simulink model "ad9361_tx_filter"  (R2021a)
settings: Solver=ode23tb  StartTime=0.0  StopTime=inf  RelTol=1e-3  EnableMultiTasking=on
PreLoadFcn:
  | ad9361_preload(bdroot,'tx')
  | Fs = 30.72e6
undefined symbols (not defined in the file or in its folder): magnitude
libraries: ad9371_utilities x1, dspmathops x1, dspsrcs4 x1, ad9361_models x1
CloseFcn:
  | clear ad9361_tx_hm1Filt ad9361_tx_hm2Filt;
  | clear ad9361_tx_hm3Filt ad9361_tx_hm4Filt;
settings Model: SimulationMode=accelerator  NumberOfSteps=100  Creator=The MathWorks Inc.  LastModifiedBy=Michael
settings SolverCC: AlgebraicLoopSolver=TrustRegion
settings DataIOCC: ExternalInput=txWaveform  SaveFormat=StructureWithTime  SaveOutput=off  SignalLogging=off  DSMLogging=off  SaveTime=off  ReturnWorkspaceOutputs=off  OutputSaveName=rx
settings OptimizationCC: DefaultParameterBehavior=Inlined  InlineInvariantSignals=on  LifeSpan=inf  SimCompilerOptimization=on
settings DebuggingCC: UnderspecifiedInitializationDetection=Classic  MergeDetectMultiDrivingBlocksExec=none  SolverPrmCheckMsg=warning  MultiTaskDSMMsg=warning  MultiTaskCondExecSysMsg=none  AllowSymbolicDim=off  SFUnexpectedBacktrackingDiag=warning  SFNoUnconditionalDefaultTransitionDiag=none  SFUndirectedBroadcastEventsDiag=none  SFExecutionAtInitializationDiag=none  SFMachineParentedDataDiag=warning  ArithmeticOperatorsInVariantConditions=warning
settings HardwareCC: ProdBitPerPointer=32  ProdBitPerSizeT=32  ProdBitPerPtrDiffT=32  ProdLargestAtomicFloat=None  ProdIntDivRoundTo=Undefined  ProdEndianess=Unspecified  ProdWordSize=32  ProdHWDeviceType=32-bit Generic
settings ModelReferenceCC: PropagateSignalLabelsOutOfModel=off
settings SFSimCC: SimUseLocalCustomCode=off  CustomCodeUndefinedFunction=UseInterfaceOnly
settings RTWCC: RTWUseLocalCustomCode=off
settings CodeAppCC: StateflowObjectComments=on
settings GRTTargetCC: TargetLangStandard=C89/C90 (ANSI)
settings ConfigComp: CovMetricSettings=dw  CovSaveCumulativeToWorkspaceVar=on  CovSaveSingleToWorkspaceVar=on  CovExternalEMLEnable=off  CovSFcnEnable=off
settings SimscapeCC: ExplicitSolverDiagnosticOptions=none  SimscapeNormalizeSystem=off

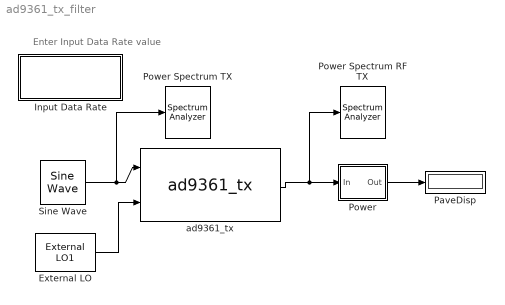
== system ad9361_tx_filter ==
  note: Enter Input Data Rate value
  External LO : ad9371_utilities/External LO1  PN=[-95 -110 -110 -125 -157]  Freq=[1e3 1e4 1e5 1e6 3e6]  PH=Random
      settings: SourceProductBaseCode=SIM_RF_TRANS
  Input Data Rate : Subsystem  mask{SampleRate=7.68e6}
      mask prompts: SampleRate "Fs"
      mask init:
      | assignin('base','Fs',SampleRate)
      mask Display: disp(['Fs = ',num2str(SampleRate)])
  PaveDisp : Display
  Power : Subsystem  mask{R=1}
      mask prompts: R "Reference Impedance [Ohm]"
      mask DialogControl DescGroupVar Prompt: Power Meter
  Power Spectrum RF TX : SpectrumAnalyzer
  Power Spectrum TX : SpectrumAnalyzer
  Sine Wave : dspsrcs4/Sine Wave  Amplitude=0.05  Frequency=3e6  Phase=0  SampleMode=Discrete  OutComplex=Complex  CompMethod=Trigonometric fcn  TableSize=Speed  SampleTime=1/Fs  SamplesPerFrame=1  ResetState=Restart at time zero  OutputFrames=off  dataType=double  wordLen=16  udDataType=sfix(16)  fracBitsMode=Best precision  numFracBits=15  OutDataTypeStr=double  LastOutDataTypeStr=double
      settings: AttributesFormatString=Sampling Rate = %<SampleTime>
  ad9361_tx : ad9361_models/ad9361_tx  TestSignal=Custom  LOFreq=2e9  Att=0  IQ_rate=7.68  RF_BW=122.88
      settings: SourceProductName=RF Blockset Models for Analog Devices RF Transceivers
  wires:
  Power/1(Out) -> PaveDisp/1
  ad9361_tx/1 -> Power/1(In), Power Spectrum RF TX/1
  Sine Wave/1 -> ad9361_tx/1, Power Spectrum TX/1
  External LO/1 -> ad9361_tx/2

== system ad9361_tx_filter/Input Data Rate ==

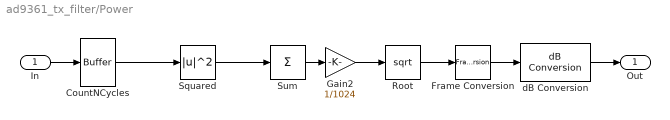
== system ad9361_tx_filter/Power ==
  In : Inport
  CountNCycles : Buffer  N=1024  OutputFrames=off
  Frame Conversion : FrameConversion  OutFrame=Sample-based
  Gain2 : Gain  Gain=1/1024
  Root : Sqrt  SaturateOnIntegerOverflow=on
  Squared : Math  Operator=magnitude^2  SignedPower=on  SaturateOnIntegerOverflow=on
  Sum : Sum  Inputs=+
  dB Conversion : dspmathops/dB Conversion  dBtype=dBm  intype=Amplitude  R=R  fuzz=on
  Out : Outport  VectorParamsAs1DForOutWhenUnconnected=off
  wires:
  dB Conversion/1 -> Out/1
  In/1 -> CountNCycles/1
  Frame Conversion/1 -> dB Conversion/1
  CountNCycles/1 -> Squared/1
  Squared/1 -> Sum/1
  Sum/1 -> Gain2/1
  Root/1 -> Frame Conversion/1
  Gain2/1 -> Root/1
